simulink model "learn02"  (R2016b)
settings: Solver=ode45  StartTime=0.0  StopTime=24  RelTol=1e-3
PreLoadFcn:
  | load('ex_househeat_measured_data.mat')
model workspace (MAT data in the model file):
  M_heater_air = 3600
  R_equivalent = 4.329e-07
  T_heater = 50
  T_roomIC = 20
  c_air = 1005.4
  m_room_air = 1470
settings Model: Creator=tapeltauer  LastModifiedBy=tapeltauer
settings DataIOCC: ExternalInput=Sheet1.getElement(1),Sheet1.getElement(2)  LoadExternalInput=on  SaveOutput=off  InspectSignalLogs=on  SaveTime=off
settings OptimizationCC: BlockReduction=off

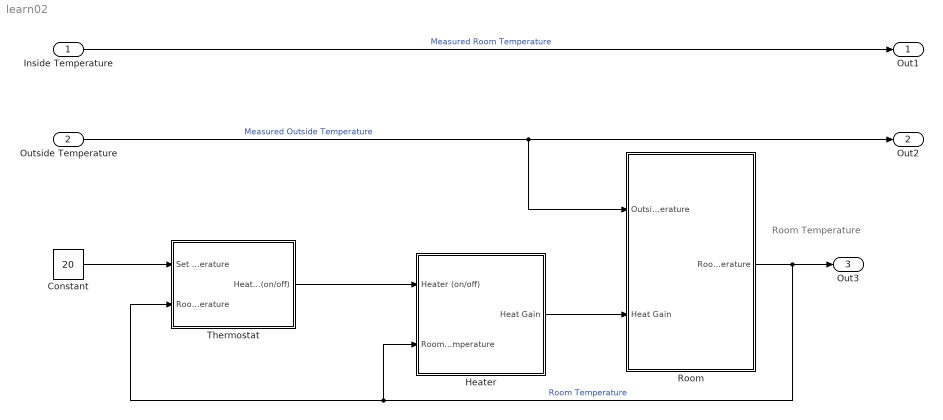
== system learn02 ==
  note: Room
      | Temperature
  Inside Temperature : Inport  Unit=°C
  Outside Temperature : Inport  Port=2  Unit=°C
  Constant : Constant  Value=20
  Heater : Subsystem
  Room : Subsystem
  Thermostat : Subsystem
  Out1 : Outport
  Out2 : Outport  Port=2  Unit=°C
  Out3 : Outport  Port=3  Unit=°C
  wires:
  Thermostat/1(Heater (on/off)) -> Heater/1(Heater (on/off))
  Heater/1(Heat Gain) -> Room/2(Heat Gain)
  Room/1(Room Temperature) -> Out3/1, Heater/2(RoomTemperature), Thermostat/2(Room Temperature)  "Room Temperature"
  Outside Temperature/1 -> Room/1(Outside Temperature), Out2/1  "Measured Outside Temperature"
  Constant/1 -> Thermostat/1(Set Room Temperature)
  Inside Temperature/1 -> Out1/1  "Measured Room Temperature"

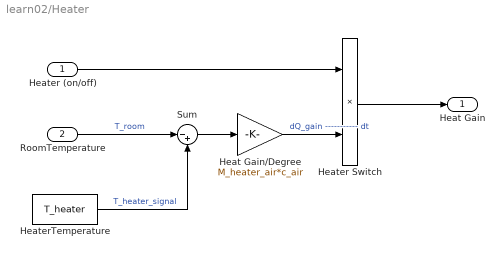
== system learn02/Heater ==
  Heater (on/off) : Inport
  RoomTemperature : Inport  Port=2
  Heat Gain/Degree : Gain  Gain=M_heater_air*c_air
  Heater Switch : Product
  HeaterTemperature : Constant  Value=T_heater
  Sum : Sum  Inputs=|-+
  Heat Gain : Outport  Unit=joule/h
  wires:
  RoomTemperature/1 -> Sum/1  "T_room"
  HeaterTemperature/1 -> Sum/2  "T_heater_signal"
  Sum/1 -> Heat Gain/Degree/1
  Heat Gain/Degree/1 -> Heater Switch/2  "dQ_gain ----------- dt"
  Heater (on/off)/1 -> Heater Switch/1
  Heater Switch/1 -> Heat Gain/1

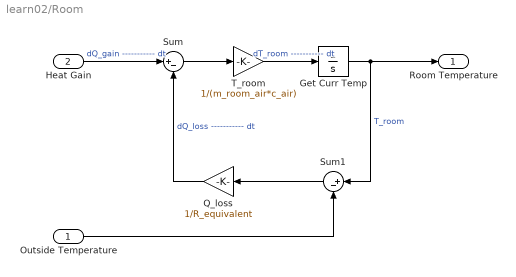
== system learn02/Room ==
  Outside Temperature : Inport
  Heat Gain : Inport  Port=2
  "Get Curr Temp " : Integrator  InitialCondition=T_roomIC
  Q_loss : Gain  Gain=1/R_equivalent
  Sum : Sum  Inputs=|+-
  Sum1 : Sum  Inputs=|+-
  T_room : Gain  Gain=1/(m_room_air*c_air)
  Room Temperature : Outport
  wires:
  Heat Gain/1 -> Sum/1  "dQ_gain ----------- dt"
  Sum/1 -> T_room/1
  T_room/1 -> "Get Curr Temp "/1  "dT_room ----------- dt"
  "Get Curr Temp "/1 -> Sum1/1, Room Temperature/1  "T_room"
  Outside Temperature/1 -> Sum1/2
  Sum1/1 -> Q_loss/1
  Q_loss/1 -> Sum/2  "dQ_loss ----------- dt"

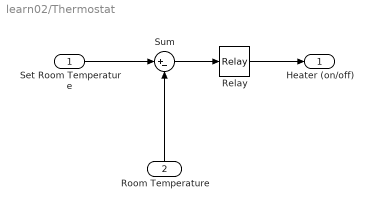
== system learn02/Thermostat ==
  Set Room Temperature : Inport
  Room Temperature : Inport  Port=2
  Relay : Relay  OnSwitchValue=0  OffSwitchValue=-5
  Sum : Sum  Inputs=|+-
  Heater (on/off) : Outport
  wires:
  Set Room Temperature/1 -> Sum/1
  Room Temperature/1 -> Sum/2
  Sum/1 -> Relay/1
  Relay/1 -> Heater (on/off)/1
